simulink model "laboratorium2_simulation"  (R2020b)
settings: Solver=FixedStepAuto  StartTime=0.0  StopTime=0.1  FixedStep=0.00001  RelTol=1e-3
values from neighbouring files (symbols this model uses):
  denominator_array = [1,1]    [laboratorium2.m]
  nominator_array = 2    [laboratorium2.m]
settings Model: Creator=student  LastModifiedBy=student

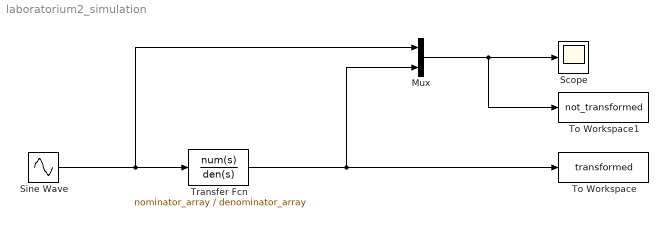
== system laboratorium2_simulation ==
  Mux : Mux  Inputs=2
  Scope : Scope
  Sine Wave : Sin  Frequency=omega (i)  SampleTime=10
  To Workspace : ToWorkspace  VariableName=transformed  SampleTime=-1
      settings: Save2DSignal=2-D array (concatenate along first dimension)
  To Workspace1 : ToWorkspace  VariableName=not_transformed  SampleTime=-1
      settings: Save2DSignal=2-D array (concatenate along first dimension)
  Transfer Fcn : TransferFcn  Numerator=nominator_array  Denominator=denominator_array
  wires:
  Sine Wave/1 -> Mux/1, Transfer Fcn/1
  Transfer Fcn/1 -> Mux/2, To Workspace/1
  Mux/1 -> To Workspace1/1, Scope/1
